simulink model "tx_system"  (R2022b)
settings: Solver=VariableStepAuto  StartTime=0.0  StopTime=10.0  RelTol=1e-3
PreLoadFcn:
  | clear;
  | OS=8
  | sample_time = 1/116e6/8;
  | 
  | carriers.LO = 22e9;
  | carriers.LOL = carriers.LO/2;
  | carriers.LOH = carriers.LO*3;
  | carriers.OUT = carriers.LO*3.5;
  | 
  | %Put all carriers in one vector for convenience
  | car_env = unique(structfun(@deal,carriers));
  | 
  | 
  | % Lower limit of frequency (governed by impulse duration):
  | Duration = sample_time*128;
  | LLFreq = 1/Duration;
  | 
  | 
  | %Upper limit of frequency (governed by sample time):
  | ULFreq = 1/(2*sample_time);
  | 
  | 
  | % Generate 1/f phase noise with -60dBc/Hz level @ 1KHz:
  | PhNoOffsets = [LLFreq 1e3 ULFreq];
  | PhNoLevels = -80-10*log10(PhNoOffsets/1e3);
  | % To extend frequency resolution down to lower frequencies,
  | % increase duration as well as the impulse response duration
  | % in the LO1 block mask
libraries: simrfV2util1 x4, simrfV2sources1 x2, dspstat3 x2, simulink x1
settings Model: SimulationMode=accelerator  Creator=hessam  LastModifiedBy=hessam

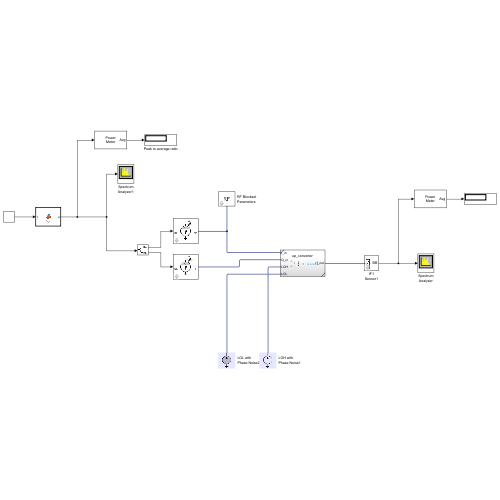
[thumbnail: Simulink's stored preview of the top-level diagram]
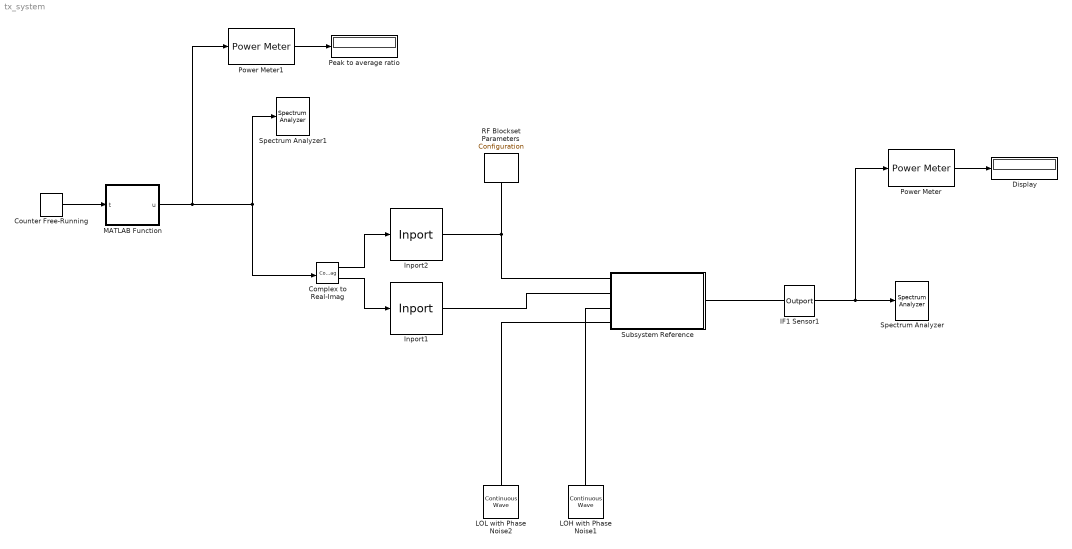
== system tx_system ==
  Complex to Real-Imag : ComplexToRealImag
  Counter Free-Running : simulink/Sources/Counter Free-Running  NumBits=24  tsamp=-1
  Display : Display
  IF1 Sensor1 : simrfV2util1/Outport  SensorType=Power  OutputFormat=Complex Baseband  CarrierFreq=carriers.OUT Hz  ZL=50  InternalGrounding=on  StepSize=-1 s  AutoStep=off
  Inport1 : simrfV2util1/Inport  SimulinkInputSignalType=Power  CarrierFreq=0 Hz  ZS=50  UseSqWave=off  NumCoeff=10  Bias=0  DutyCyc=50  InternalGrounding=on
  Inport2 : simrfV2util1/Inport  SimulinkInputSignalType=Power  CarrierFreq=0 Hz  ZS=50  UseSqWave=off  NumCoeff=10  Bias=0  DutyCyc=50  InternalGrounding=on
  LOH with Phase Noise1 : simrfV2sources1/Continuous Wave  CWSourceType=Ideal voltage  Z0=0  IVoltage=1 V  ICurrent=0 A  MagPower=0 W  QVoltage=0 V  QCurrent=0 A  AnglePower=0  CarrierFreq=carriers.LOH Hz  AddPhaseNoise=off  PhaseNoiseOffset=PhNoOffsets  PhaseNoiseLevel=PhNoLevels  AutoImpulseLength=on  ImpulseLength=1e-10 s  InternalGrounding=on
  LOL with Phase Noise2 : simrfV2sources1/Continuous Wave  CWSourceType=Ideal voltage  Z0=0  IVoltage=1 V  ICurrent=0 A  MagPower=0 W  QVoltage=0 V  QCurrent=0 A  AnglePower=0  CarrierFreq=carriers.LOL Hz  AddPhaseNoise=on  PhaseNoiseOffset=PhNoOffsets  PhaseNoiseLevel=PhNoLevels  AutoImpulseLength=on  ImpulseLength=1e-10 s  InternalGrounding=on
  MATLAB Function : MATLAB Function  TreatAsAtomicUnit=on
  Peak to average ratio : Display
  Power Meter : dspstat3/Power Meter  Measurement=Average power  ReferenceLoad=1  OutputPowerUnits=dBm  WindowLength=256  OverlapLength=255  AllowArbitraryInputLength=on  ComputeCCDF=off  PowerRange=50  PowerResolution=0.1  CCDFOutput=Relative power (dB above average power)  ProbabilityVector=[ 10; 1; 0.1; 0.01; 0.001; 0.0001 ]  RelativePowerVector=[ 0; 3; 6; 9; 12 ]  ResetPort=off  SimulateUsing=Code generation
      settings: LibrarySourceBlock=commutil2/Power Meter
  Power Meter1 : dspstat3/Power Meter  Measurement=Average power  ReferenceLoad=1  OutputPowerUnits=dBm  WindowLength=256  OverlapLength=255  AllowArbitraryInputLength=on  ComputeCCDF=off  PowerRange=50  PowerResolution=0.1  CCDFOutput=Relative power (dB above average power)  ProbabilityVector=[ 10; 1; 0.1; 0.01; 0.001; 0.0001 ]  RelativePowerVector=[ 0; 3; 6; 9; 12 ]  ResetPort=off  SimulateUsing=Code generation
      settings: LibrarySourceBlock=commutil2/Power Meter
  RF Blockset Parameters : simrfV2util1/Configuration  AutoFreq=on  Tones="[11  66] GHz"  Harmonics="[5  5]"  NormalizeCarrierPower=on  SolverType=Auto  UseCCode=on  StepSize=sample_time s  AddNoise=off  defaultRNG=on  Seed=0  Temperature=293.15 K  SolverDelFlag=0  AbsTol=1e-6  RelTol=1e-3  MaxIter=10  ErrorEstimationType=2-norm over all variables  EnableInterpFilter=off  HiddenFIRfilterControllerParam=off  SmallSignalApprox=off  AllSimFreqs=on  SimFreqs=[] Hz  SimFreqsInternal=[]  SamplesPerFrame=1
  Spectrum Analyzer : SpectrumAnalyzer
  Spectrum Analyzer1 : SpectrumAnalyzer
  Subsystem Reference : Subsystem  ReferencedSubsystem=up_converter
      settings: PortSchema="{\"entries\":[{\"content\":{\"sides\":[{\"content\":{\"connectorIds\":[\"LConn3\",\"LConn4\",\"LConn2\",\"LConn1\"]},\"type\":\"ConnectorPlacement.EquallySpacedRectSide\",\"uuid\":\"13d4ea5a-fa0b-40a2-b728-0cb27c04c45c\"},{\"content\":{\"connectorIds\":[\"LConn5\"],\"side\":\"RIGHT\"},\"type\":\"ConnectorPlacement.EquallySpacedRectSide\",\"uuid\":\"f63a5880-6d48-44cf-a00e-69a0a1f06c9f\"},{\"content\":{\"connectorIds\":[],\"side\":\"TOP\"},\"type\":\"ConnectorPlacement.EquallySpacedRectSide\",\"uuid\":\"0624c078-97eb-4241-acb3-cf6a765df704\"}]},\"type\":\"ConnectorPlacement.EquallySpacedConnector\",\"uuid\":\"a841a9cc-0770-4745-91fc-8b3b1f9434fa\"}],\"packageUris\":[\"http://schema.mathworks.com/mf0/Connector/R2020b\"],\"version\":\"1.0\"}"
  wires:
  Counter Free-Running/1 -> MATLAB Function/1(t)
  MATLAB Function/1(u) -> Power Meter1/1, Spectrum Analyzer1/1, Complex to Real-Imag/1
  Power Meter/1 -> Display/1
  Power Meter1/1 -> Peak to average ratio/1
  Complex to Real-Imag/1 -> Inport2/1
  Complex to Real-Imag/2 -> Inport1/1
  IF1 Sensor1/1 -> Power Meter/1, Spectrum Analyzer/1
  connections:
  Subsystem Reference/LConn1 -- LOL with Phase Noise2/LConn1
  LOH with Phase Noise1/LConn1 -- Subsystem Reference/LConn2
  Subsystem Reference/LConn3 -- RF Blockset Parameters/LConn1 -- Inport2/RConn1
  Subsystem Reference/LConn4 -- Inport1/RConn1
  IF1 Sensor1/LConn1 -- Subsystem Reference/LConn5

== matlab function tx_system/MATLAB Function ==
  data: u output; t input
function u   = fcn(t)
   %test of the block
   t=double(t);
   pdb=-3;   %dial input power in dBm 50-ohm reference
   v = sqrt(1/1000*10^(pdb/10));
   f=[1 2 3 4 5 6  ]*455e-5;
   u=v*sum(exp(2.0*3.14*f*t*1j));
